simulink model "LQR_Control_diagram"  (R2014b)
settings: Solver=ode45  StartTime=0.0  StopTime=10.0  RelTol=1e-3
values from neighbouring files (symbols this model uses):
  Klqr_continuous = lqr(A,B,Qx,Qu)    [main.m]
  Kr_continuous = pinv(D - (C - D*Klqr_continuous)*(A - B*Klqr_continuous)\B)    [main.m]
  r = [0 0 0 0 0 0 0 0 0 0 0 0]'    [main.m]
  u_op = operating_voltage    [main.m]
undefined symbols (not defined in the file or in its folder): Xo
settings Model: Creator=Abhiram  LastModifiedBy=gunnar

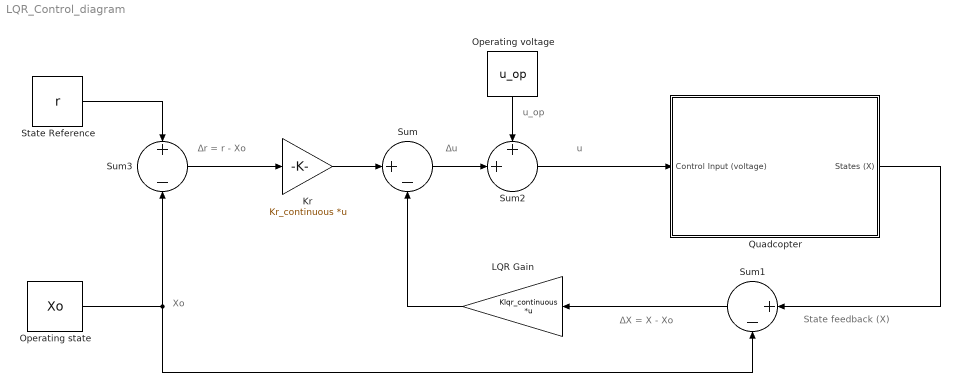
== system LQR_Control_diagram ==
  note: Xo
  note: u
  note: Δr = r - Xo
  note: u_op
  note: ΔX = X - Xo
  note: State feedback (X)
  note: Δu
  Kr : Gain  Gain=Kr_continuous  Multiplication=Matrix(K*u)
  LQR Gain : Gain  Gain=Klqr_continuous  Multiplication=Matrix(K*u)
  Operating state : Constant  Value=Xo  VectorParams1D=off
  Operating voltage : Constant  Value=u_op  VectorParams1D=off
  Quadcopter : Subsystem
  State Reference : Constant  Value=r  VectorParams1D=off
  Sum : Sum  Inputs=|+-
  Sum1 : Sum  Inputs=|+-
  Sum2 : Sum  Inputs=++|
  Sum3 : Sum  Inputs=+|-
  wires:
  Sum2/1 -> Quadcopter/1(Control Input (voltage))
  Sum1/1 -> LQR Gain/1
  Kr/1 -> Sum/1
  LQR Gain/1 -> Sum/2
  Sum/1 -> Sum2/2
  Operating voltage/1 -> Sum2/1
  Sum3/1 -> Kr/1
  State Reference/1 -> Sum3/1
  Operating state/1 -> Sum1/2, Sum3/2
  Quadcopter/1(States (X)) -> Sum1/1

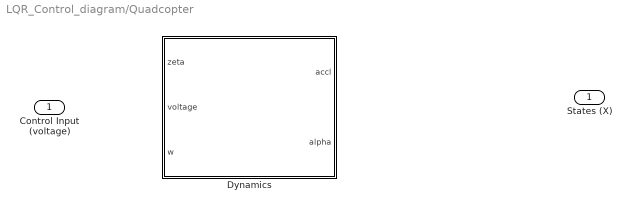
== system LQR_Control_diagram/Quadcopter ==
  Control Input (voltage) : Inport
  Dynamics : MATLAB Function  TreatAsAtomicUnit=on
  States (X) : Outport

== matlab function LQR_Control_diagram/Quadcopter/Dynamics ==
  data: zeta input; voltage input; accl output; alpha output; w input
function [accl, alpha] = fcn(zeta, voltage, w)

    Ixx = 2.09*10^(-05);
    Iyy = 2.09*10^(-05);
    Izz = 3.81*10^(-05);
    I = diag([Ixx,Iyy,Izz]);                              % Inertia matrix - needs revision

    d = 0.046;
    m = 0.027;
    g = 9.8;

%%%%%%%%%%%%%%%%%%%%%%%%%%%%%%%%%%%%%%%%%%%%%%%%%%%%%%%%%%%%%%%%%%%%%%%%%%%
%3
    theta = zeta(1);         % pitch    
    phi = zeta(2);           % roll
    psi = zeta(3);           % yaw  
    
% %     omega_square = [omega(1)^2 omega(2)^2 omega(3)^2 omega(4)^2]';
% %     T_b = C*omega_square;    
% %     %     C = [Ct     Ct    Ct    Ct;
% %     %          0      d*Ct  0     -d*Ct;
% %     %         -d*Ct   0     d*Ct  0;
% %     %         -Cq     Cq   -Cq    Cq ]; % Plus config
    
    [T_b] = thrust(voltage);              % non linear function for thrust
    
    F_e = T_b(1)*[-sin(theta); cos(theta)*sin(phi); cos(theta)*cos(phi)];
    
    Tau_e = [T_b(2) T_b(3) T_b(4)]';
    G = [0 0 m*g]';
% G = [0 0 0]';

    T_e = [F_e - G; Tau_e];

    I_a = [m*eye(3)    zeros(3,3);
           zeros(3,3)         I ];

    w_cross = cross(w,I*w);

    % Needs Revision
    A = I_a \ ( T_e - [0;0;0;w_cross] );
    
    accl = A(1:3);
    alpha = A(4:6);

end
